simulink model "Simulink_Funktionsblock"  (R2019b)
settings: Solver=VariableStepAuto  StartTime=0.0  StopTime=600  RelTol=1e-3
values from neighbouring files (symbols this model uses):
  Par_Ini = [1000;293.15;293.15]    [INIT_Nachbrenner.m]    (also in INIT_Startbrenner.m = [293.15;293.15;293.15]; Modellbildung_Brenner.m = [293.15;293.15;293.15]; matlab_workspace.mat = [293.15 293.15 293.15])
  u_AP = [ms_wt_f]    [INIT_Nachbrenner.m]    (also in INIT_Startbrenner.m = [ms_bg ; ms_wt_f ]; Modellbildung_Brenner.m = [ T_bg_in ; T_wt_in ; T_u ; ms_bg ; ms_wt_f ]; matlab_workspace.mat = [293.15 293.15 293.15 0.000724954280964 0.0045])
  vec_par = zeros(23,1)    [INIT_Nachbrenner.m]    (also in INIT_Startbrenner.m; Modellbildung_Brenner.m = zeros(19,1); matlab_workspace.mat = [0.000724954280964 1060.66142274 1060.66142274 0.02624391402)
settings Model: Creator=mh981  LastModifiedBy=nikitavetter
settings DataIOCC: ReturnWorkspaceOutputs=off
settings DebuggingCC: ArithmeticOperatorsInVariantConditions=warning
settings SFSimCC: CustomCodeUndefinedFunction=UseInterfaceOnly

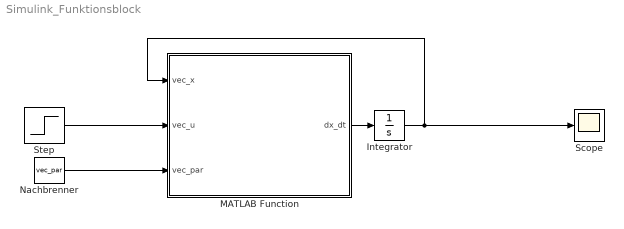
== system Simulink_Funktionsblock ==
  Integrator : Integrator  InitialCondition=Par_Ini
  MATLAB Function : MATLAB Function  TreatAsAtomicUnit=on
  Nachbrenner : Constant  Value=vec_par
  Scope : Scope
  Step : Step  Time=2  Before=u_AP  After=u_AP  SampleTime=0
  wires:
  MATLAB Function/1(dx_dt) -> Integrator/1
  Integrator/1 -> MATLAB Function/1(vec_x), Scope/1
  Step/1 -> MATLAB Function/2(vec_u)
  Nachbrenner/1 -> MATLAB Function/3(vec_par)

== matlab function Simulink_Funktionsblock/MATLAB Function ==
  data: vec_x input; vec_u input; dx_dt output; vec_par input
%#eml
function dx_dt = Modell_simulink(vec_x ,vec_u , vec_par)

dx_dt = Modellgleichung (vec_x ,vec_u , vec_par);
